simulink model "project3_week_1"  (R2020b)
settings: Solver=VariableStepAuto  StartTime=0.0  StopTime=10.0  RelTol=1e-3
settings Model: Creator=RASIKA MALGI  LastModifiedBy=RASIKA MALGI

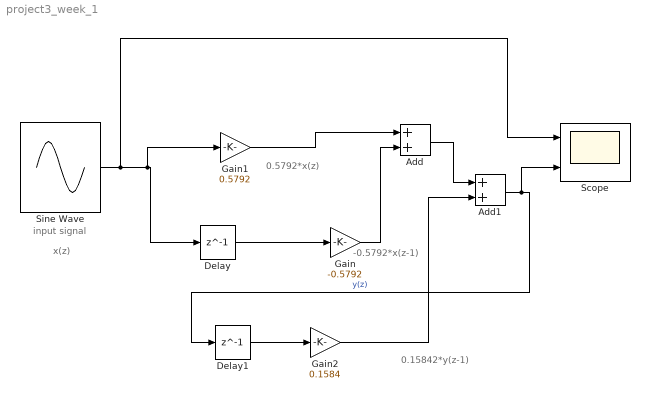
== system project3_week_1 ==
  note: 0.15842*y(z-1)
  note: -0.5792*x(z-1)
  note: 0.5792*x(z)
  note: x(z)
  note: input signal
  Add : Sum
  Add1 : Sum
  Delay : Delay  DelayLength=1  InitialCondition=0
  Delay1 : Delay  DelayLength=1  InitialCondition=0
  Gain : Gain  Gain=-0.5792
  Gain1 : Gain  Gain=0.5792
  Gain2 : Gain  Gain=0.1584
  Scope : Scope  NumInputPorts=2
  Sine Wave : Sin  SampleTime=0
  wires:
  Sine Wave/1 -> Gain1/1, Delay/1, Scope/1
  Delay/1 -> Gain/1
  Gain/1 -> Add/2
  Gain1/1 -> Add/1
  Delay1/1 -> Gain2/1
  Add/1 -> Add1/1
  Gain2/1 -> Add1/2
  Add1/1 -> Scope/2, Delay1/1  "y(z)"
